simulink model "RCAMDemo_Interface"  (R2021a)
settings: Solver=ode45  StartTime=0.0  StopTime=simulation.t_final  RelTol=1e-3  EnableMultiTasking=on
libraries: UWAerospaceBlockset_Animation x3, aerolibfltsims x2, aerolibanimutils x1
settings Model: Creator=lum  LastModifiedBy=chris
settings SolverCC: AlgebraicLoopSolver=TrustRegion
settings DataIOCC: LimitDataPoints=on  SaveFormat=Array  ReturnWorkspaceOutputs=off
settings OptimizationCC: ExpressionDepthLimit=2147483647  LifeSpan=inf
settings DebuggingCC: UnderspecifiedInitializationDetection=Classic  MergeDetectMultiDrivingBlocksExec=none  SolverPrmCheckMsg=warning  FcnCallInpInsideContextMsg=warning  StateNameClashWarn=warning  SFUnexpectedBacktrackingDiag=warning  SFNoUnconditionalDefaultTransitionDiag=warning  SFExecutionAtInitializationDiag=none  SFMachineParentedDataDiag=warning  ArithmeticOperatorsInVariantConditions=warning
settings HardwareCC: ProdBitPerPointer=32  ProdBitPerSizeT=32  ProdBitPerPtrDiffT=32  ProdLargestAtomicFloat=None  ProdIntDivRoundTo=Undefined  ProdEndianess=Unspecified  ProdWordSize=32  ProdHWDeviceType=32-bit Generic
settings ModelReferenceCC: PropagateSignalLabelsOutOfModel=off
settings SFSimCC: SimUseLocalCustomCode=off  CustomCodeUndefinedFunction=UseInterfaceOnly
settings RTWCC: RTWUseLocalCustomCode=off
settings CodeAppCC: StateflowObjectComments=on
settings GRTTargetCC: TargetLangStandard=C89/C90 (ANSI)  CombineOutputUpdateFcns=off  GRTInterface=on
settings ConfigComp: CovMetricSettings=dw  CovSaveCumulativeToWorkspaceVar=on  CovSaveSingleToWorkspaceVar=on  CovExternalEMLEnable=off  CovSFcnEnable=off

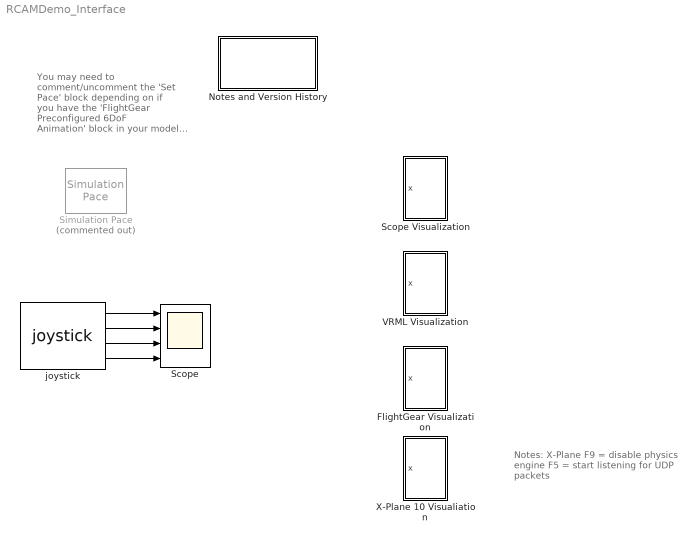
== system RCAMDemo_Interface ==
  note: You may need to comment/uncomment the 'Set Pace' block depending on if you have the 'FlightGear Preconfigured 6DoF Animation' block in your model or not.
  note: Notes:
      | X-Plane
      | F9 = disable physics engine
      | F5 = start listening for UDP packets
  FlightGear Visualization : Subsystem
  Notes and Version History : Subsystem
  Scope : Scope  NumInputPorts=4
  Scope Visualization : Subsystem
  Simulation Pace : aerolibanimutils/Simulation Pace  Commented=on  SimulationPace=1  SleepMode=Auto  OutputPaceError=off  SampleTime=1/30
  VRML Visualization : Subsystem
  X-Plane 10 Visualiation : Subsystem
  joystick : UWAerospaceBlockset_Animation/joystick  joystickID=Joystick2  max_aileron_deflection=30*pi/180  max_elevator_deflection=20*pi/180  max_rudder_deflection=20*pi/180  sample_time=simulation.sample_time
  wires:
  joystick/2 -> Scope/2
  joystick/1 -> Scope/1
  joystick/3 -> Scope/3
  joystick/4 -> Scope/4

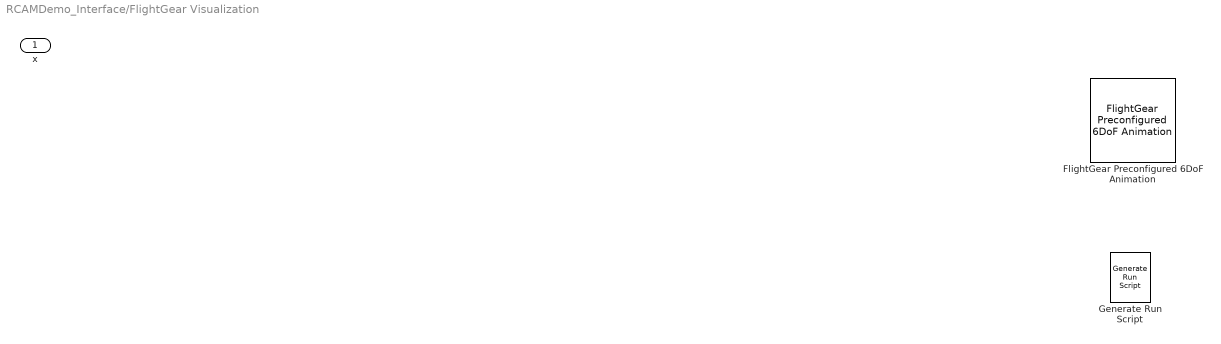
== system RCAMDemo_Interface/FlightGear Visualization ==
  x : Inport
  FlightGear Preconfigured 6DoF Animation : aerolibfltsims/FlightGear Preconfigured 6DoF Animation  xFlightGearVersion=v2018.1  DestinationIpAddress=127.0.0.1  DestinationPort=5502  SampleTime=1/30  packetVersion=24
  Generate Run Script : aerolibfltsims/Generate Run Script  Architecture=Win64  dataFlow=Send  GeometryModelName=c172p  AirportId=KSFO  RunwayId=10L  InitialAltitude=7224  InitialHeading=113  OffsetDistance=4.72  OffsetAzimuth=0  InstallScenery=off  DisableShaders=on  OriginAddress=127.0.0.1  DestinationPort=5502  OriginPort=5505  LocalAddress=127.0.0.1  OutputFileName=runfg.bat  FlightGearBaseDirectory=C:\Program Files\FlightGear 2018.1.1

== system RCAMDemo_Interface/Notes and Version History ==
  note: A subset of files that can be released to students to support the final project.
      |
      | Christopher Lum
      | lum@uw.edu
      |
      | Version History
      | 03/28/20: Updated to Matlab R2018b
      | 04/09/20: Removed blocks to make this a minimal set of files that can be released to students
      | 03/08/22: Added FlightGear visualization

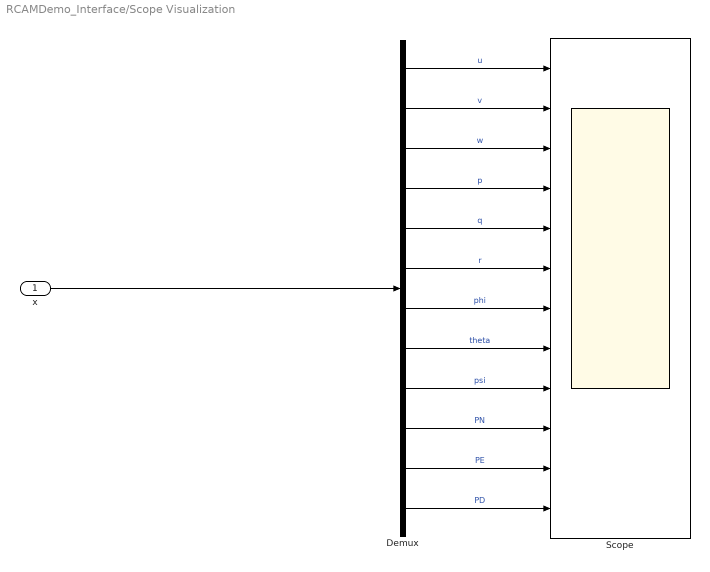
== system RCAMDemo_Interface/Scope Visualization ==
  x : Inport
  Demux : Demux  Outputs=12
  Scope : Scope  NumInputPorts=12
  wires:
  Demux/12 -> Scope/12  "PD"
  Demux/11 -> Scope/11  "PE"
  Demux/10 -> Scope/10  "PN"
  Demux/9 -> Scope/9  "psi"
  Demux/8 -> Scope/8  "theta"
  Demux/7 -> Scope/7  "phi"
  Demux/6 -> Scope/6  "r"
  Demux/5 -> Scope/5  "q"
  Demux/1 -> Scope/1  "u"
  Demux/4 -> Scope/4  "p"
  Demux/2 -> Scope/2  "v"
  Demux/3 -> Scope/3  "w"
  x/1 -> Demux/1

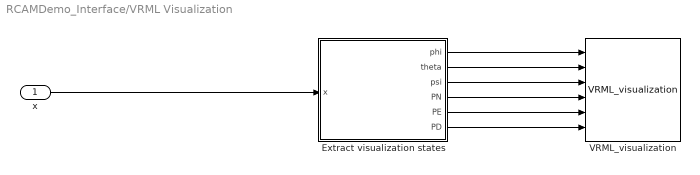
== system RCAMDemo_Interface/VRML Visualization ==
  x : Inport
  Extract visualization states : Subsystem
  VRML_visualization : UWAerospaceBlockset_Animation/VRML_visualization
  wires:
  Extract visualization states/2(theta) -> VRML_visualization/2
  Extract visualization states/1(phi) -> VRML_visualization/1
  Extract visualization states/5(PE) -> VRML_visualization/5
  Extract visualization states/6(PD) -> VRML_visualization/6
  Extract visualization states/4(PN) -> VRML_visualization/4
  Extract visualization states/3(psi) -> VRML_visualization/3
  x/1 -> Extract visualization states/1(x)

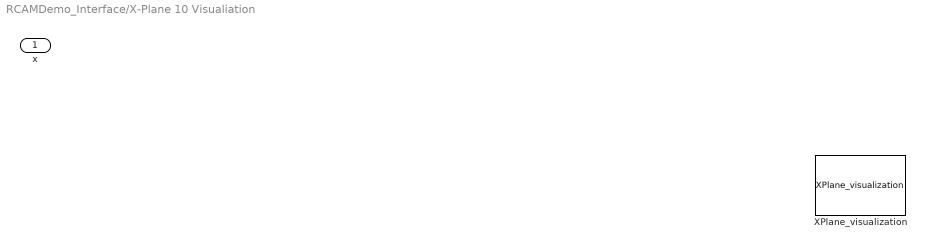
== system RCAMDemo_Interface/X-Plane 10 Visualiation ==
  x : Inport
  XPlane_visualization : UWAerospaceBlockset_Animation/XPlane_visualization  IP_address=simulation.x_plane.state_visualization.IP_address  plugin_listening_port_number=simulation.x_plane.state_visualization.plugin_listening_port_number  numDigitsOfPrecision=simulation.x_plane.state_visualization.numDigitsOfPrecision

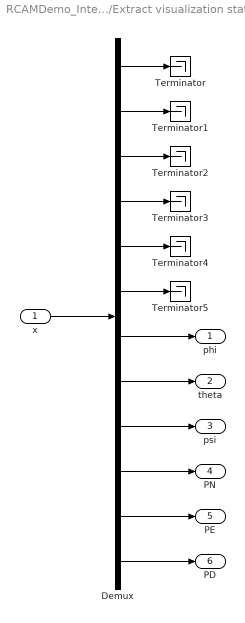
== system RCAMDemo_Interface/VRML Visualization/Extract visualization states ==
  x : Inport
  Demux : Demux  Outputs=12
  Terminator{,1..5} (6 alike) : Terminator
  phi : Outport  VectorParamsAs1DForOutWhenUnconnected=off
  theta : Outport  Port=2  VectorParamsAs1DForOutWhenUnconnected=off
  psi : Outport  Port=3  VectorParamsAs1DForOutWhenUnconnected=off
  PN : Outport  Port=4  VectorParamsAs1DForOutWhenUnconnected=off
  PE : Outport  Port=5  VectorParamsAs1DForOutWhenUnconnected=off
  PD : Outport  Port=6  VectorParamsAs1DForOutWhenUnconnected=off
  wires:
  x/1 -> Demux/1
  Demux/1 -> Terminator/1
  Demux/2 -> Terminator1/1
  Demux/3 -> Terminator2/1
  Demux/4 -> Terminator3/1
  Demux/5 -> Terminator4/1
  Demux/6 -> Terminator5/1
  Demux/7 -> phi/1
  Demux/8 -> theta/1
  Demux/9 -> psi/1
  Demux/10 -> PN/1
  Demux/11 -> PE/1
  Demux/12 -> PD/1
